simulink model "Advanced_SmartMotor_Blocks_18b"  (R2018b)
settings: Solver=FixedStepAuto  StartTime=0.0  StopTime=inf  RelTol=1e-3
settings Model: SimulationMode=external  Creator=avenkata  LastModifiedBy=josea
settings DataIOCC: ReturnWorkspaceOutputs=on
settings OptimizationCC: EnhancedBackFolding=on  PassReuseOutputArgsAs=Individual arguments  MaxStackSize=64  OptimizeBlockOrder=speed  DifferentSizesBufferReuse=on  OptimizationCustomize=off
settings DebuggingCC: ParameterTunabilityLossMsg=error  SymbolicDimsDataTypeCodeGenerationDiagnostic=none
settings HardwareCC: ProdBitPerPointer=32  ProdBitPerSizeT=32  ProdBitPerPtrDiffT=32  ProdLargestAtomicInteger=Long  ProdLargestAtomicFloat=Double  ProdWordSize=32  ProdHWDeviceType=ARM Compatible->ARM Cortex  UseEmbeddedCoderFeatures=off
settings SFSimCC: MATLABDynamicMemAlloc=off
settings RTWCC: SystemTargetFile=ert.tlc  HardwareBoard=VEX V5 Robot Brain  TLCOptions="-aInlineSetEventsForThisBaseRateFcn=TLC_FALSE -aSuppressMultiTaskScheduler=TLC_FALSE  -aRateBasedStepFcn=0"  TemplateMakefile=ert_default_tmf  GenerateReport=on  Toolchain=GNU Tools for ARM Embedded Processors  IncludeHyperlinkInReport=on  LaunchReport=on  GenerateTraceInfo=on  GenerateTraceReport=on  GenerateTraceReportSl=on  GenerateTraceReportSf=on  GenerateTraceReportEml=on
settings CodeAppCC: ForceParamTrailComments=on  IgnoreCustomStorageClasses=off  OperatorAnnotations=on  SimulinkDataObjDesc=on  SFDataObjDesc=on  InsertBlockDesc=on
settings ERTTargetCC: SupportNonInlinedSFcns=on  ExtMode=on

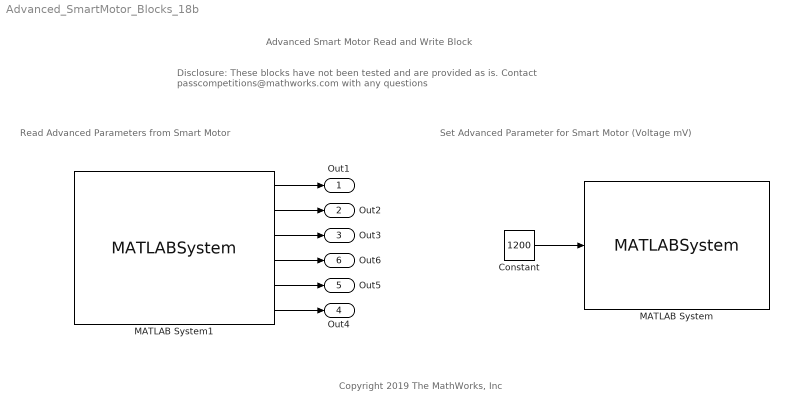
== system Advanced_SmartMotor_Blocks_18b ==
  note: Disclosure: These blocks have not been tested and are provided as is. Contact passcompetitions@mathworks.com with any questions
  note: Advanced Smart Motor Read and Write Block
  note: Set Advanced Parameter for Smart Motor (Voltage mV)
  note: Read Advanced Parameters from Smart Motor
  note: Copyright 2019 The MathWorks, Inc
  Constant : Constant  Value=1200  SampleTime=-1
  MATLAB System : MATLABSystem  System=Advanced_SmartMotorWrite  motorPort=1  scaleFactor=6:1  MotorBrakeMode=Coast  OperationMode=Advanced Control
      mask Type: Advanced_SmartMotorWrite
      mask Display:
      | color('white');
      | plot([100,100,100,100]*1,[100,100,100,100]*1);
      | plot([100,100,100,100]*0,[100,100,100,100]*0);
      | color('black');
      | image(fullfile(codertarget.vexv5.internal.getSpPkgRootDir, 'resources', 'vex-v5-motor2.png'),'center');
      | patch([0.8, 0.8, 1, 1], [0.82857, 1, 1, 0.82857], [1, 1, 1]);
      | color('blue');
      | text(99, 92, 'VEX V5 ', 'horizontalAlignment', 'right');
      | color('black');
      | text(62,12,'Port: 1','horizontalAlignment','center');
      | 
      | port_label('Input',1,'Voltage(mV)');
  MATLAB System1 : MATLABSystem  System=Advanced_SmartMotorRead  motorPort=1  additionalOutput=off  SampleTime=0.02
      mask Type: Advanced_SmartMotorRead
      mask Display:
      | color('white');
      | plot([100,100,100,100]*1,[100,100,100,100]*1);
      | plot([100,100,100,100]*0,[100,100,100,100]*0);
      | color('black');
      | image(fullfile(codertarget.vexcommon.internal.getRootDir, 'resources', 'encoder.jpg'),'center');
      | patch([0.8, 0.8, 1, 1], [0.82857, 1, 1, 0.82857], [1, 1, 1]);
      | color('blue');
      | text(75, 92, 'VEX V5 ', 'horizontalAlignment', 'right');
      | color('black');
      | text(50,15,'Port: 1','horizontalAlignment','center');
      | 
      | 
      | port_label('output',1,'Voltage');
      | port_label('output',2,'Current');
      | port_label('output',3,'Power');
      | port_label('output',4,'Torque');
      | port_label('output',5,'Efficiency');
      | port_label('output',6,'Temperature');
  Out1 : Outport
  Out2 : Outport  Port=2
  Out3 : Outport  Port=3
  Out4 : Outport  Port=4
  Out5 : Outport  Port=5
  Out6 : Outport  Port=6
  wires:
  Constant/1 -> MATLAB System/1
  MATLAB System1/1 -> Out1/1
  MATLAB System1/2 -> Out2/1
  MATLAB System1/6 -> Out4/1
  MATLAB System1/5 -> Out5/1
  MATLAB System1/4 -> Out6/1
  MATLAB System1/3 -> Out3/1
